simulink model "MotorPropModel"  (R2019b)
settings: Solver=VariableStepAuto  StartTime=0.0  StopTime=inf  FixedStep=1/  RelTol=1e-3
values from neighbouring files (symbols this model uses):
  Jl = 6.01e-5    (= 6.01e-05)    [loadSystemVariables.m]
  Jm = 996e-6    (= 0.000996)    [loadSystemVariables.m]
  Kb = (1/1000)*9.5493    (= 0.0095493)    [loadSystemVariables.m]
  Kf = 1    [loadSystemVariables.m]
  Kk = 1e4    (= 10000)    [loadSystemVariables.m]
  Km = 0.5    [loadSystemVariables.m]
  Kt = 18.16e-3    (= 0.01816)    [loadSystemVariables.m]
  Kv = 1000    [loadSystemVariables.m]
  L = series(P,G)    [SISO_phi.m]    (also in SISO_x.m; basicSISO_phi.m; basicSISO_x.m; basicSISO_y.m)
  R = 0.256    [loadSystemVariables.m]
  s = qctrl(0,[],1)    [SISO_phi.m]    (also in SISO_x.m; basicSISO_phi.m; basicSISO_x.m; basicSISO_y.m)
undefined symbols (not defined in the file or in its folder): DiscIntNeverNeededParam
libraries: cstblocks x4
settings Model: Creator=Iftah  LastModifiedBy=Iftah

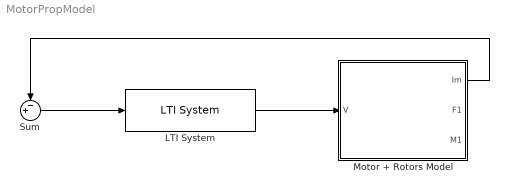
== system MotorPropModel ==
  LTI System : cstblocks/LTI System  sys=c2d(1/(tf(s)+1),1/1024)  IC=[]
  Motor + Rotors Model : Subsystem
  Sum : Sum  Inputs=-+|
  wires:
  Sum/1 -> LTI System/1
  LTI System/1 -> Motor + Rotors Model/1(V)
  Motor + Rotors Model/1(Im) -> Sum/1

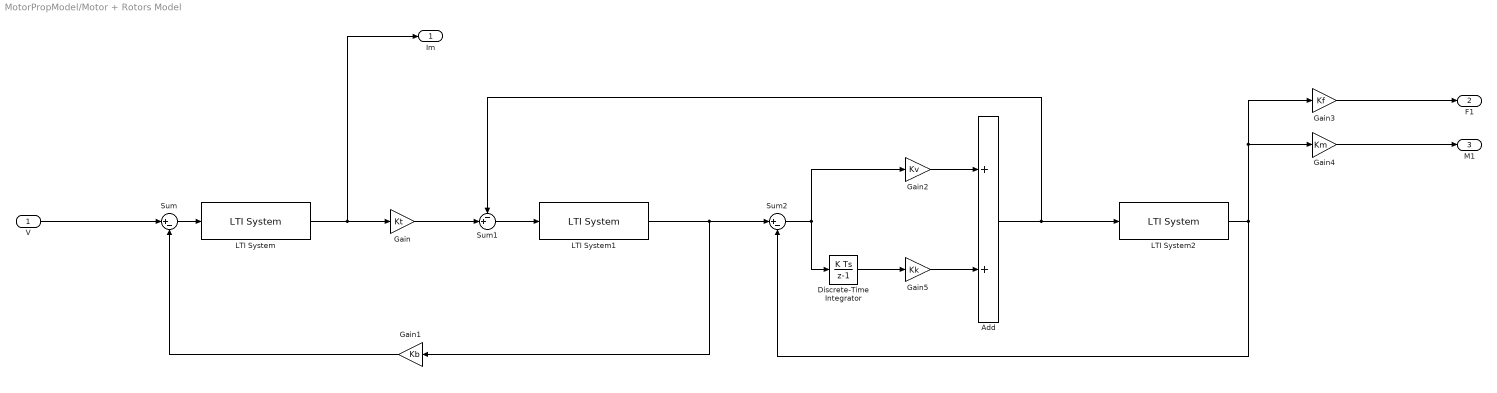
== system MotorPropModel/Motor + Rotors Model ==
  V : Inport
  Add : Sum
  Discrete-Time Integrator : DiscreteIntegrator  SampleTime=1/1024  ICPrevOutput=DiscIntNeverNeededParam  ICPrevScaledInput=DiscIntNeverNeededParam
  Gain : Gain  Gain=Kt
  Gain1 : Gain  Gain=Kb
  Gain2 : Gain  Gain=Kv
  Gain3 : Gain  Gain=Kf
  Gain4 : Gain  Gain=Km
  Gain5 : Gain  Gain=Kk
  LTI System : cstblocks/LTI System  sys=c2d(1/(L*tf(s)+R),1/1024)  IC=[]
  LTI System1 : cstblocks/LTI System  sys=c2d(1/(Jm*tf(s)),1/1024)  IC=[]
  LTI System2 : cstblocks/LTI System  sys=c2d(1/(Jl*tf(s)),1/1024)  IC=[]
  Sum : Sum  Inputs=|+-
  Sum1 : Sum  Inputs=-+|
  Sum2 : Sum  Inputs=|+-
  Im : Outport
  F1 : Outport  Port=2
  M1 : Outport  Port=3
  wires:
  V/1 -> Sum/1
  LTI System/1 -> Im/1, Gain/1
  LTI System1/1 -> Sum2/1, Gain1/1
  Sum/1 -> LTI System/1
  Gain1/1 -> Sum/2
  Gain/1 -> Sum1/2
  Sum1/1 -> LTI System1/1
  Sum2/1 -> Discrete-Time Integrator/1, Gain2/1
  Gain2/1 -> Add/1
  Gain5/1 -> Add/2
  Add/1 -> LTI System2/1, Sum1/1
  LTI System2/1 -> Sum2/2, Gain3/1, Gain4/1
  Gain3/1 -> F1/1
  Gain4/1 -> M1/1
  Discrete-Time Integrator/1 -> Gain5/1
